simulink model "Four_Degrees_of_Freedom_Model_of_Car_Vibration"  (R2023a)
settings: Solver=VariableStepAuto  StartTime=0.0  StopTime=10.0  RelTol=1e-3
values from neighbouring files (symbols this model uses):
  a = 1.26    [siziyouduxiangyingdama.m]
  b = 1.53    [siziyouduxiangyingdama.m]
  cf = 1450    [siziyouduxiangyingdama.m]
  cr = 1450    [siziyouduxiangyingdama.m]
  I = 1910    [siziyouduxiangyingdama.m]
  kf = 17500    [siziyouduxiangyingdama.m]
  kr = 22500    [siziyouduxiangyingdama.m]
  ktf = 322340    [siziyouduxiangyingdama.m]
  ktr = 493000    [siziyouduxiangyingdama.m]
  ms = 1815    [siziyouduxiangyingdama.m]
  muf = 51.5    [siziyouduxiangyingdama.m]
  mur = 49.5    [siziyouduxiangyingdama.m]
libraries: simulink x1
settings Model: Creator=dell  LastModifiedBy=JiangXin
settings SolverCC: AlgebraicLoopSolver=TrustRegion
settings DataIOCC: ReturnWorkspaceOutputs=off
settings DebuggingCC: UnconnectedInputMsg=warning  UnconnectedOutputMsg=warning  UnconnectedLineMsg=warning  ArithmeticOperatorsInVariantConditions=warning
settings ModelReferenceCC: EnableRefExpFcnMdlSchedulingChecks=on
settings SFSimCC: SimUseLocalCustomCode=off  CustomCodeUndefinedFunction=UseInterfaceOnly
settings RTWCC: RTWUseLocalCustomCode=off
settings CodeAppCC: StateflowObjectComments=on

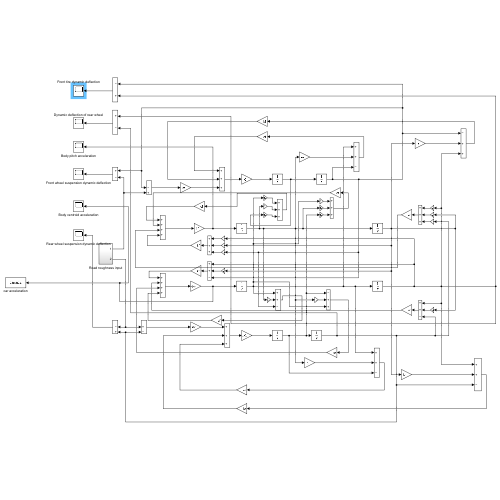
[thumbnail: Simulink's stored preview of the top-level diagram]
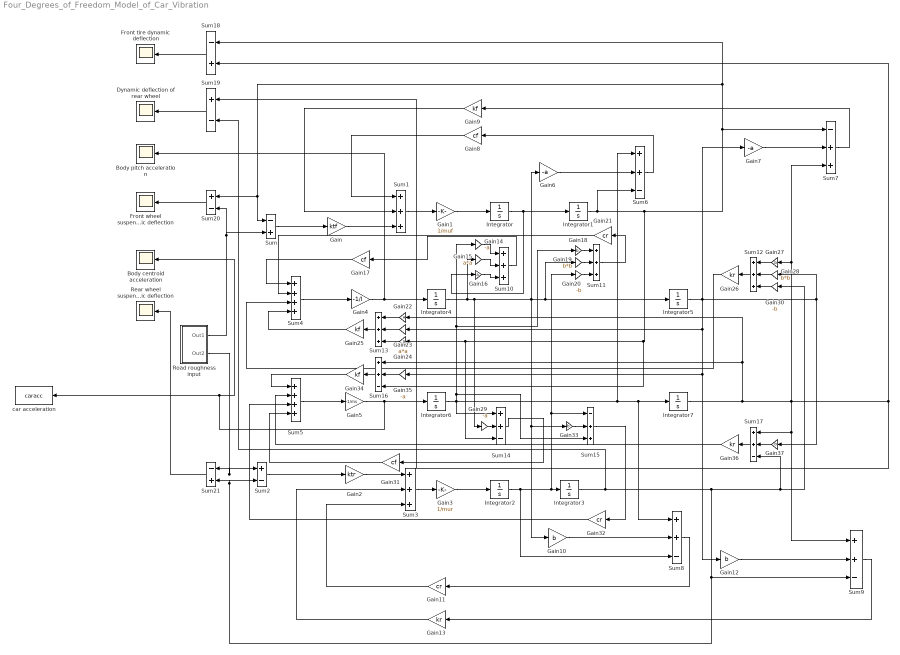
== system Four_Degrees_of_Freedom_Model_of_Car_Vibration ==
  "Body centroid acceleration " : Scope
  Body pitch acceleration : Scope
  Dynamic deflection of rear wheel : Scope
  Front tire dynamic deflection : Scope
  Front wheel suspension dynamic deflection : Scope
  Gain : Gain  Gain=ktf
  Gain1 : Gain  Gain=1/muf
  Gain{10,12,18,27,33,37} (6 alike) : Gain  Gain=b
  Gain11 : Gain  Gain=cr
  Gain13 : Gain  Gain=kr
  Gain{6..7,14,29,35} (5 alike) : Gain  Gain=-a
  Gain15 : Gain  Gain=a*a
  Gain16 : Gain  Gain=a
  Gain17 : Gain  Gain=cf
  Gain19 : Gain  Gain=b*b
  Gain2 : Gain  Gain=ktr
  Gain20 : Gain  Gain=-b
  Gain21 : Gain  Gain=cr
  Gain22 : Gain  Gain=a
  Gain23 : Gain  Gain=a*a
  Gain24 : Gain  Gain=a
  Gain25 : Gain  Gain=kf
  Gain26 : Gain  Gain=kr
  Gain28 : Gain  Gain=b*b
  Gain3 : Gain  Gain=1/mur
  Gain30 : Gain  Gain=-b
  Gain31 : Gain  Gain=cf
  Gain32 : Gain  Gain=cr
  Gain34 : Gain  Gain=kf
  Gain36 : Gain  Gain=kr
  Gain4 : Gain  Gain=-1/I
  Gain5 : Gain  Gain=-1/ms
  Gain8 : Gain  Gain=cf
  Gain9 : Gain  Gain=kf
  Integrator{,1..7} (8 alike) : Integrator
  Rear wheel suspension dynamic deflection : Scope
  Road roughness input : Subsystem
  Sum : Sum  Inputs=|-+
  Sum{1,3,10..13} (6 alike) : Sum  Inputs=+++
  Sum{6,8..9,14,16..17} (6 alike) : Sum  Inputs=++-
  Sum15 : Sum  Inputs=-++
  Sum18 : Sum  Inputs=-+
  Sum19 : Sum  Inputs=+-
  Sum2 : Sum  Inputs=|+-
  Sum20 : Sum  Inputs=+-
  Sum21 : Sum  Inputs=|-+
  Sum4 : Sum  Inputs=++++
  Sum5 : Sum  Inputs=++++
  Sum7 : Sum  Inputs=-++
  car acceleration : ToWorkspace  VariableName=caracc  SaveFormat=Timeseries  SampleTime=-1
  wires:
  Road roughness input/1(Out1) -> Sum20/2, Sum/2
  Sum/1 -> Gain/1
  Sum1/1 -> Gain1/1
  Gain1/1 -> Integrator/1
  Integrator/1 -> Gain16/1, Integrator1/1
  Integrator1/1 -> Sum16/3, Sum14/3, Gain24/1, Sum18/1, Sum20/1, Sum/1, Sum7/1, Sum6/3
  Road roughness input/2(Out2) -> Sum21/1, Sum2/1
  Sum2/1 -> Gain2/1
  Sum3/1 -> Gain3/1
  Gain3/1 -> Integrator2/1
  Integrator2/1 -> Sum8/3, Sum15/1, Gain20/1, Integrator3/1
  Sum4/1 -> Gain4/1
  Gain4/1 -> Body pitch acceleration/1, Integrator4/1
  Integrator4/1 -> Gain15/1, Gain29/1, Gain10/1, Gain33/1, Gain6/1, Gain19/1, Integrator5/1
  Sum5/1 -> Gain5/1
  Integrator6/1 -> Sum8/1, Integrator7/1, Sum6/1, Gain18/1, Gain14/1, Sum15/3, Sum14/1
  Gain6/1 -> Sum6/2
  Gain/1 -> Sum1/3
  Integrator7/1 -> Sum19/1, Sum18/2, Sum17/1, Sum9/1, Gain27/1, Sum7/3, Sum16/1, Gain22/1
  Gain7/1 -> Sum7/2
  Sum6/1 -> Gain8/1
  Gain8/1 -> Sum1/1
  Sum7/1 -> Gain9/1
  Gain9/1 -> Sum1/2
  Gain10/1 -> Sum8/2
  Sum8/1 -> Gain11/1
  Gain2/1 -> Sum3/1
  Gain11/1 -> Sum3/3
  Gain12/1 -> Sum9/2
  Sum9/1 -> Gain13/1
  Gain13/1 -> Sum3/2
  Gain14/1 -> Sum10/1
  Gain15/1 -> Sum10/2
  Gain16/1 -> Sum10/3
  Sum10/1 -> Gain17/1
  Gain17/1 -> Sum4/1
  Gain18/1 -> Sum11/1
  Gain19/1 -> Sum11/2
  Gain20/1 -> Sum11/3
  Sum11/1 -> Gain21/1
  Gain21/1 -> Sum4/2
  Gain22/1 -> Sum13/1
  Gain23/1 -> Sum13/2
  Gain24/1 -> Sum13/3
  Sum13/1 -> Gain25/1
  Gain25/1 -> Sum4/4
  Sum12/1 -> Gain26/1
  Gain26/1 -> Sum4/3
  Gain27/1 -> Sum12/1
  Gain28/1 -> Sum12/2
  Gain30/1 -> Sum12/3
  Gain29/1 -> Sum14/2
  Sum14/1 -> Gain31/1
  Gain31/1 -> Sum5/4
  Sum15/1 -> Gain32/1
  Gain32/1 -> Sum5/3
  Gain33/1 -> Sum15/2
  Sum16/1 -> Gain34/1
  Gain34/1 -> Sum5/1
  Gain35/1 -> Sum16/2
  Integrator5/1 -> Gain23/1, Gain35/1, Gain12/1, Gain37/1, Gain28/1, Gain7/1
  Sum17/1 -> Gain36/1
  Gain36/1 -> Sum5/2
  Gain37/1 -> Sum17/2
  Sum18/1 -> Front tire dynamic deflection/1
  Sum19/1 -> Dynamic deflection of rear wheel/1
  Sum20/1 -> Front wheel suspension dynamic deflection/1
  Sum21/1 -> Rear wheel suspension dynamic deflection/1
  Integrator3/1 -> Sum17/3, Gain30/1, Sum9/3, Sum21/2, Sum2/2, Sum19/2
  Gain5/1 -> car acceleration/1, "Body centroid acceleration "/1, Integrator6/1

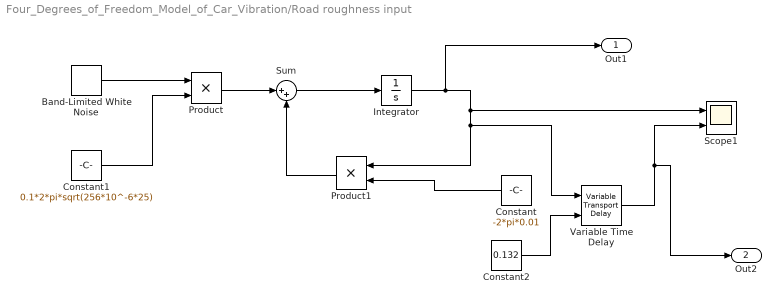
== system Four_Degrees_of_Freedom_Model_of_Car_Vibration/Road roughness input ==
  Band-Limited White Noise : simulink/Sources/Band-Limited White Noise  Cov=[0.25]  Ts=0.01  seed=[23531]
  Constant : Constant  Value=-2*pi*0.01
  Constant1 : Constant  Value=0.1*2*pi*sqrt(256*10^-6*25)
  Constant2 : Constant  Value=0.132
  Integrator : Integrator
  Product : Product
  Product1 : Product
  Scope1 : Scope  NumInputPorts=2
  Sum : Sum  Inputs=|++
  Variable Time Delay : VariableTransportDelay  MaximumDelay=10
  Out1 : Outport  VectorParamsAs1DForOutWhenUnconnected=off
  Out2 : Outport  Port=2  VectorParamsAs1DForOutWhenUnconnected=off
  wires:
  Product/1 -> Sum/1
  Band-Limited White Noise/1 -> Product/1
  Sum/1 -> Integrator/1
  Integrator/1 -> Out1/1, Scope1/1, Variable Time Delay/1, Product1/1
  Variable Time Delay/1 -> Scope1/2, Out2/1
  Constant2/1 -> Variable Time Delay/2
  Constant/1 -> Product1/2
  Product1/1 -> Sum/2
  Constant1/1 -> Product/2
